simulink model "Park"  (R2014b)
settings: Solver=ode45  StartTime=0.0  StopTime=0.1  RelTol=1e-3
libraries: powerlib_meascontrol x1
settings Model: Creator=Lei  LastModifiedBy=Lei

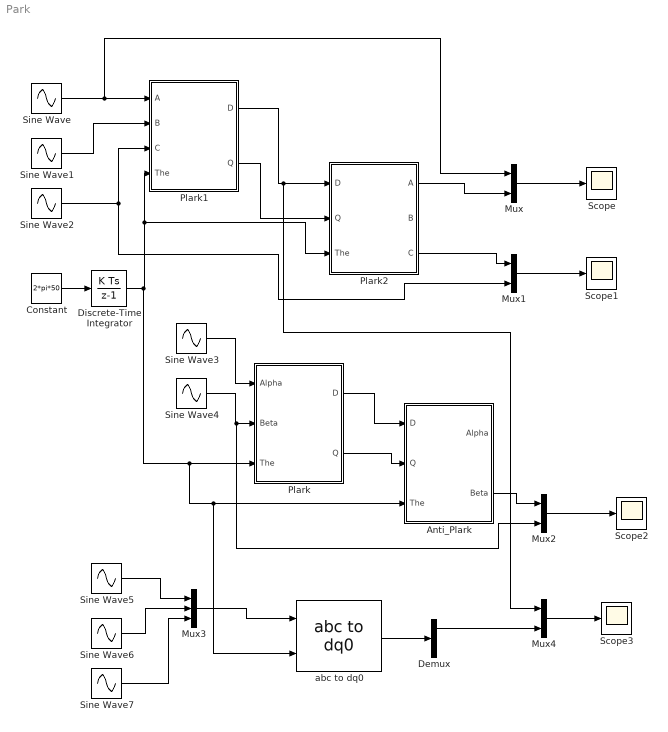
== system Park ==
  Anti_Plark : Subsystem
  Constant : Constant  Value=2*pi*50
  Demux : Demux  Outputs=3
  Discrete-Time Integrator : DiscreteIntegrator  InitialConditionSetting=State (most efficient)  SampleTime=10e-6
  Mux{,1..2,4} (4 alike) : Mux  Inputs=2
  Mux3 : Mux  Inputs=3
  Plark : Subsystem
  Plark1 : Subsystem
  Plark2 : Subsystem
  Scope{,1..3} (4 alike) : Scope
      Scope settings: YMin=-150  YMax=150
      Scope1 settings: ShowLegends=on  YMin=-150  YMax=150
      Scope2 settings: ShowLegends=on  YMin=-150  YMax=150  SaveName=ScopeData2
      Scope3 settings: ShowLegends=on  YMin=-150  YMax=150  SaveName=ScopeData3
  Sine Wave : Sin  Amplitude=100  Frequency=2*pi*50  SampleTime=10e-6
  Sine Wave1 : Sin  Amplitude=100  Frequency=2*pi*50  Phase=-2/3*pi  SampleTime=10e-6
  Sine Wave2 : Sin  Amplitude=100  Frequency=2*pi*50  Phase=2/3*pi  SampleTime=10e-6
  Sine Wave3 : Sin  Amplitude=100  Frequency=2*pi*50  SampleTime=10e-6
  Sine Wave4 : Sin  Amplitude=100  Frequency=2*pi*50  Phase=pi/2  SampleTime=10e-6
  Sine Wave5 : Sin  Amplitude=100  Frequency=2*pi*50  SampleTime=10e-6
  Sine Wave6 : Sin  Amplitude=100  Frequency=2*pi*50  Phase=-2/3*pi  SampleTime=10e-6
  Sine Wave7 : Sin  Amplitude=100  Frequency=2*pi*50  Phase=2/3*pi  SampleTime=10e-6
  abc to dq0 : powerlib_meascontrol/Transformations/abc to dq0  Alignment=Aligned with phase A axis
  wires:
  Plark1/1(D) -> Mux4/1, Plark2/1(D)
  Plark1/2(Q) -> Plark2/2(Q)
  Sine Wave1/1 -> Plark1/2(B)
  Constant/1 -> Discrete-Time Integrator/1
  Discrete-Time Integrator/1 -> abc to dq0/2, Anti_Plark/3(The), Plark/3(The), Plark2/3(The), Plark1/4(The)
  Mux/1 -> Scope/1
  Plark2/1(A) -> Mux/2
  Sine Wave/1 -> Mux/1, Plark1/1(A)
  Plark2/3(C) -> Mux1/1
  Sine Wave2/1 -> Plark1/3(C), Mux1/2
  Mux1/1 -> Scope1/1
  Plark/2(Q) -> Anti_Plark/2(Q)
  Sine Wave4/1 -> Mux2/2, Plark/2(Beta)
  Sine Wave3/1 -> Plark/1(Alpha)
  Mux2/1 -> Scope2/1
  Anti_Plark/2(Beta) -> Mux2/1
  Sine Wave5/1 -> Mux3/1
  Sine Wave6/1 -> Mux3/2
  Sine Wave7/1 -> Mux3/3
  Mux3/1 -> abc to dq0/1
  abc to dq0/1 -> Demux/1
  Demux/1 -> Mux4/2
  Plark/1(D) -> Anti_Plark/1(D)
  Mux4/1 -> Scope3/1

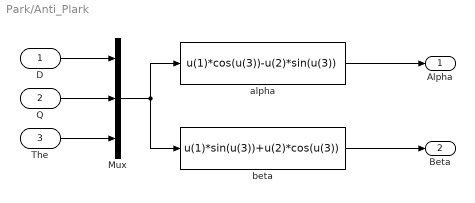
== system Park/Anti_Plark ==
  D : Inport
  Q : Inport  Port=2
  The : Inport  Port=3
  Mux : Mux  Inputs=3
  alpha : Fcn  Expr=u(1)*cos(u(3))-u(2)*sin(u(3))
  beta : Fcn  Expr=u(1)*sin(u(3))+u(2)*cos(u(3))
  Alpha : Outport
  Beta : Outport  Port=2
  wires:
  alpha/1 -> Alpha/1
  Q/1 -> Mux/2
  The/1 -> Mux/3
  D/1 -> Mux/1
  Mux/1 -> beta/1, alpha/1
  beta/1 -> Beta/1

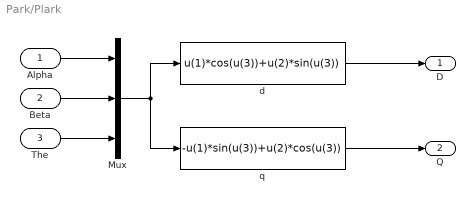
== system Park/Plark ==
  Alpha : Inport
  Beta : Inport  Port=2
  The : Inport  Port=3
  Mux : Mux  Inputs=3
  d : Fcn  Expr=u(1)*cos(u(3))+u(2)*sin(u(3))
  q : Fcn  Expr=-u(1)*sin(u(3))+u(2)*cos(u(3))
  D : Outport
  Q : Outport  Port=2
  wires:
  d/1 -> D/1
  Beta/1 -> Mux/2
  The/1 -> Mux/3
  Alpha/1 -> Mux/1
  Mux/1 -> q/1, d/1
  q/1 -> Q/1

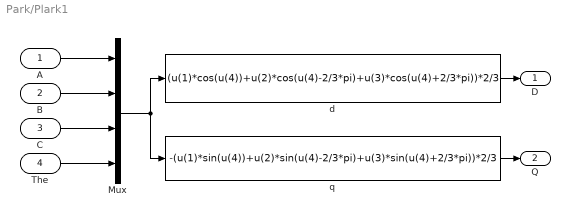
== system Park/Plark1 ==
  A : Inport
  B : Inport  Port=2
  C : Inport  Port=3
  The : Inport  Port=4
  Mux : Mux
  d : Fcn  Expr=(u(1)*cos(u(4))+u(2)*cos(u(4)-2/3*pi)+u(3)*cos(u(4)+2/3*pi))*2/3
  q : Fcn  Expr=-(u(1)*sin(u(4))+u(2)*sin(u(4)-2/3*pi)+u(3)*sin(u(4)+2/3*pi))*2/3
  D : Outport
  Q : Outport  Port=2
  wires:
  Mux/1 -> q/1, d/1
  A/1 -> Mux/1
  B/1 -> Mux/2
  d/1 -> D/1
  The/1 -> Mux/4
  C/1 -> Mux/3
  q/1 -> Q/1

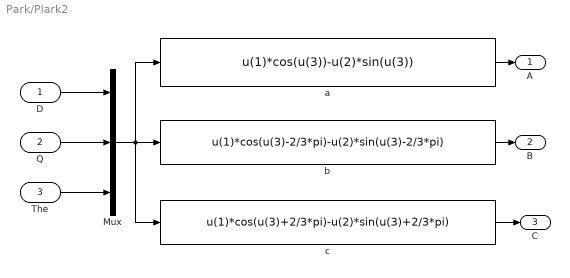
== system Park/Plark2 ==
  D : Inport
  Q : Inport  Port=2
  The : Inport  Port=3
  Mux : Mux  Inputs=3
  a : Fcn  Expr=u(1)*cos(u(3))-u(2)*sin(u(3))
  b : Fcn  Expr=u(1)*cos(u(3)-2/3*pi)-u(2)*sin(u(3)-2/3*pi)
  c : Fcn  Expr=u(1)*cos(u(3)+2/3*pi)-u(2)*sin(u(3)+2/3*pi)
  A : Outport
  B : Outport  Port=2
  C : Outport  Port=3
  wires:
  b/1 -> B/1
  The/1 -> Mux/3
  a/1 -> A/1
  D/1 -> Mux/1
  Q/1 -> Mux/2
  Mux/1 -> c/1, a/1, b/1
  c/1 -> C/1
